simulink model "try_again_agin"  (R2025a)
settings: Solver=VariableStepAuto  StartTime=0.0  StopTime=inf  FixedStep=1e-5  MaxStep=1e-4  RelTol=1e-3
values from neighbouring files (symbols this model uses):
  B = 0.0001    [main.m]
  init_Thetar = 0    [main.m]
  init_Thetar_tilde = -3*pi/7    (= -1.34639685154)    [main.m]
  Is_rated = 10    [main.m]
  J = 0.045    [main.m]
  Kas = 1/Kps    (= 3.05577490736)    [main.m]
  Kic = Rs*Wcc    (= 1256.63706144)    [main.m]
  Kis = J*Wsc^2/5/Kt    (= 2.05616758356)    [main.m]
  Kpc = Lds*Wcc    (= 18.8495559215)    [main.m]
  Kps = J*Wsc/Kt    (= 0.327249234749)    [main.m]
  Lamf = 0.12    [main.m]
  Lds = 30.0e-3    (= 0.03)    [main.m]
  Lqs = 40.0e-3    (= 0.04)    [main.m]
  mm = 2    [main.m]
  Mode = 2    [main.m]
  P = 24    [main.m]
  Rs = 2    [main.m]
  V_inj = 60    [main.m]
  w_h = 2*pi*800    (= 5026.54824574)    [main.m]
settings Model: Creator=moon  LastModifiedBy=moon
settings RTWCC: GPUComputeCapability=3.5

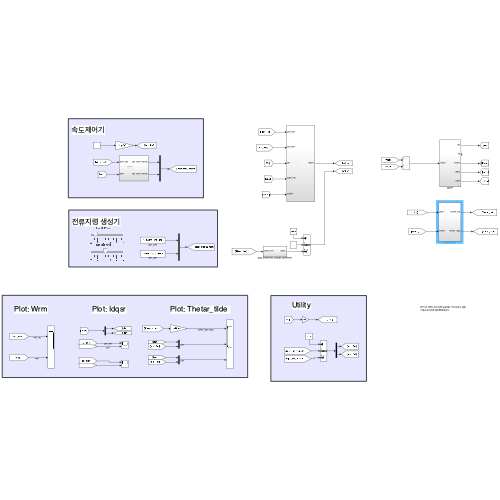
[thumbnail: Simulink's stored preview of the top-level diagram]
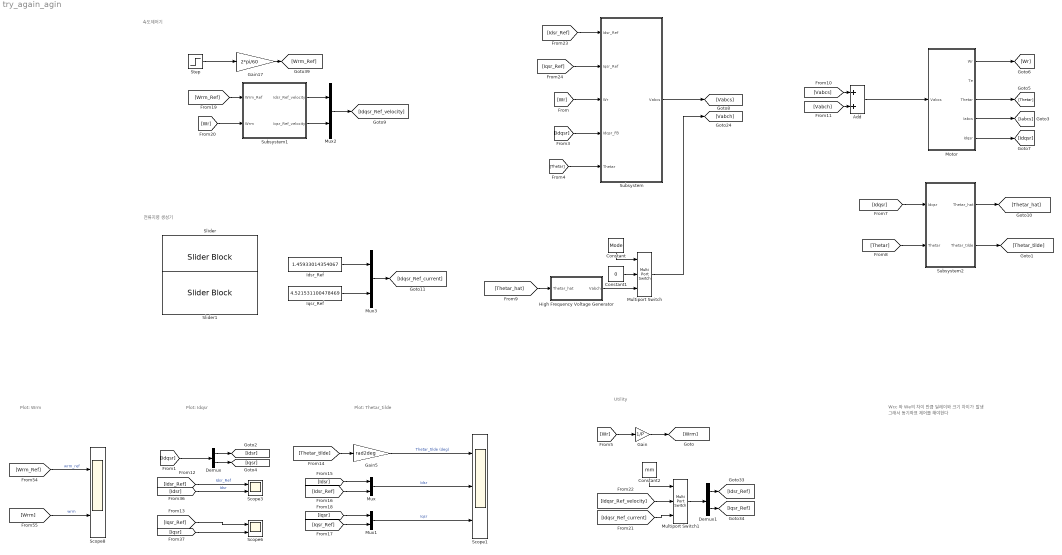
== system try_again_agin ==
  note: Plot: Thetar_tilde
  note: 전류지령 생성기
  note: 속도제어기
  note: 그래서 동기좌표 제어를 해야한다
  note: Wcc 와 We의 차이 만큼 딜레이와 크기 차이가 발생
  note: Plot: Wrm
  note: Plot: Idqsr
  note: Utility
  Add : Sum
  Constant : Constant  Value=Mode
  Constant1 : Constant  Value=0
  Constant2 : Constant  Value=mm
  Demux : Demux  Outputs=2
  Demux1 : Demux  Outputs=2
  Gain : Gain  Gain=1/P
  Gain17 : Gain  Gain=2*pi/60
  Gain5 : Gain  Gain=rad2deg
  High Frequency Voltage Generator : Subsystem
  Idsr_Ref : Constant  Value=1.45933014354067
  Iqsr_Ref : Constant  Value=4.521531100478469
  Motor : Subsystem
  Multiport Switch : MultiPortSwitch  Inputs=2  SaturateOnIntegerOverflow=off  InputSameDT=off
  Multiport Switch1 : MultiPortSwitch  Inputs=2  SaturateOnIntegerOverflow=off  InputSameDT=off
  Mux{,1..3} (4 alike) : Mux  Inputs=2
  Scope1 : Scope  NumInputPorts=3
      settings: ActiveDisplayYMinimum=-5.1750271088581092  ActiveDisplayYMaximum=6.5752439797229876  DataLoggingVariableName=ScopeData8
  Scope3 : Scope  NumInputPorts=2
      settings: ActiveDisplayYMinimum=-1  ActiveDisplayYMaximum=1  DataLoggingVariableName=ScopeData4
  Scope6 : Scope  NumInputPorts=2
      settings: ActiveDisplayYMinimum=-1.0209344961629327  ActiveDisplayYMaximum=9.1884104654663972  DataLoggingVariableName=ScopeData5
  Scope8 : Scope  NumInputPorts=2
      settings: ActiveDisplayYMinimum=-124.203723618037  ActiveDisplayYMaximum=1117.8335125623332
  Slider : SliderBlock  ScaleMax=10
  Slider1 : SliderBlock  ScaleMax=10
  Step : Step  After=200  SampleTime=0
  Subsystem : Subsystem
  Subsystem1 : Subsystem
  Subsystem2 : Subsystem
  wires:
  [Wrm_Ref] -> Scope8/1  "wrm_ref"
  [Wrm] -> Scope8/2  "wrm"
  Gain17/1 -> [Wrm_Ref]
  Step/1 -> Gain17/1
  Motor/4(Iabcs) -> [Iabcs]
  Motor/3(Thetar) -> [Thetar]
  Motor/1(Wr) -> [Wr]
  Add/1 -> Motor/1(Vabcs)
  Motor/5(Idqsr) -> [Idqsr]
  [Wr] -> Subsystem/3(Wr)
  [Idqsr] -> Subsystem/4(Idqsr_FB)
  Subsystem/1(Vabcs) -> [Vabcs]
  [Thetar] -> Subsystem/5(Thetar)
  [Wr] -> Gain/1
  Gain/1 -> [Wrm]
  [Idqsr] -> Subsystem2/1(Idqsr)
  [Thetar] -> Subsystem2/2(Thetar)
  Subsystem2/1(Thetar_hat) -> [Thetar_hat]
  Subsystem2/2(Thetar_tilde) -> [Thetar_tilde]
  [Thetar_hat] -> High Frequency Voltage Generator/1(Thetar_hat)
  High Frequency Voltage Generator/1(Vabch) -> Multiport Switch/3
  Constant1/1 -> Multiport Switch/2
  Constant/1 -> Multiport Switch/1
  [Vabch] -> Add/2
  [Vabcs] -> Add/1
  Multiport Switch/1 -> [Vabch]
  [Idsr_Ref] -> Scope3/1  "Idsr_Ref"
  [Iqsr] -> Scope6/2
  [Idsr] -> Scope3/2  "Idsr"
  [Iqsr_Ref] -> Scope6/1
  [Idqsr] -> Demux/1
  Demux/1 -> [Idsr]
  Demux/2 -> [Iqsr]
  [Idsr] -> Mux/1
  Mux/1 -> Scope1/2  "Idsr"
  Mux1/1 -> Scope1/3  "Iqsr"
  [Idsr_Ref] -> Mux/2
  Gain5/1 -> Scope1/1  "Thetar_tilde (deg)"
  [Iqsr] -> Mux1/1
  [Thetar_tilde] -> Gain5/1
  [Wrm_Ref] -> Subsystem1/1(Wrm_Ref)
  [Wr] -> Subsystem1/2(Wrm)
  Subsystem1/1(Idsr_Ref_velocity) -> Mux2/1
  Subsystem1/2(Iqsr_Ref_velocity) -> Mux2/2
  Mux2/1 -> [Idqsr_Ref_velocity]
  Iqsr_Ref/1 -> Mux3/2
  Idsr_Ref/1 -> Mux3/1
  Mux3/1 -> [Idqsr_Ref_current]
  Constant2/1 -> Multiport Switch1/1
  [Idqsr_Ref_velocity] -> Multiport Switch1/2
  [Idqsr_Ref_current] -> Multiport Switch1/3
  Multiport Switch1/1 -> Demux1/1
  Demux1/1 -> [Idsr_Ref]
  Demux1/2 -> [Iqsr_Ref]
  [Idsr_Ref] -> Subsystem/1(Idsr_Ref)
  [Iqsr_Ref] -> Subsystem/2(Iqsr_Ref)
  [Iqsr_Ref] -> Mux1/2

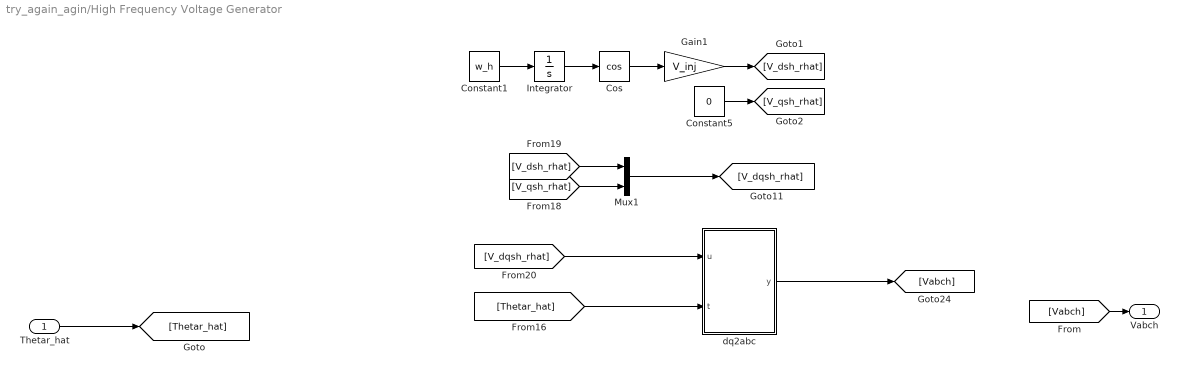
== system try_again_agin/High Frequency Voltage Generator ==
  Thetar_hat : Inport
  Constant1 : Constant  Value=w_h
  Constant5 : Constant  Value=0
  Cos : Trigonometry  Operator=cos
  Gain1 : Gain  Gain=V_inj
  Integrator : Integrator
  Mux1 : Mux  Inputs=2
  dq2abc : MATLAB Function  TreatAsAtomicUnit=on
  Vabch : Outport
  wires:
  Constant5/1 -> [V_qsh_rhat]
  Integrator/1 -> Cos/1
  Constant1/1 -> Integrator/1
  Mux1/1 -> [V_dqsh_rhat]
  Gain1/1 -> [V_dsh_rhat]
  dq2abc/1(y) -> [Vabch]
  [Thetar_hat] -> dq2abc/2(t)
  Cos/1 -> Gain1/1
  [V_dsh_rhat] -> Mux1/1
  [V_qsh_rhat] -> Mux1/2
  [V_dqsh_rhat] -> dq2abc/1(u)
  [Vabch] -> Vabch/1
  Thetar_hat/1 -> [Thetar_hat]

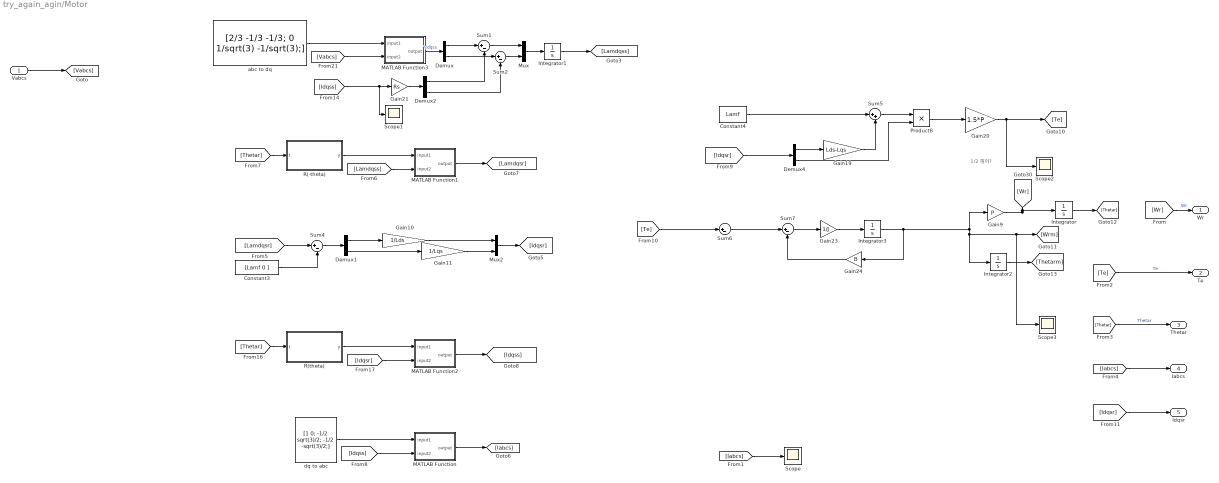
== system try_again_agin/Motor ==
  note: 1/2 해야?
  Vabcs : Inport
  Constant3 : Constant  Value=[Lamf 0 ]
  Constant4 : Constant  Value=Lamf
  Demux{,1..2,4} (4 alike) : Demux  Outputs=2
  Gain10 : Gain  Gain=1/Lds
  Gain11 : Gain  Gain=1/Lqs
  Gain19 : Gain  Gain=Lds-Lqs
  Gain20 : Gain  Gain=1.5*P
  Gain21 : Gain  Gain=Rs
  Gain23 : Gain  Gain=1/J
  Gain24 : Gain  Gain=B
  Gain9 : Gain  Gain=P
  Integrator : Integrator  InitialCondition=init_Thetar
  Integrator1 : Integrator
  Integrator2 : Integrator
  Integrator3 : Integrator
  MATLAB Function : MATLAB Function  TreatAsAtomicUnit=on
  MATLAB Function1 : MATLAB Function  TreatAsAtomicUnit=on
  MATLAB Function2 : MATLAB Function  TreatAsAtomicUnit=on
  MATLAB Function3 : MATLAB Function  TreatAsAtomicUnit=on
  Mux : Mux  Inputs=2
  Mux2 : Mux  Inputs=2
  Product8 : Product
  R(-theta) : Subsystem
      mask Display: image(imread('img/rotateInverseMatrix.png'))
  R(theta) : Subsystem
      mask Display: image(imread('img/rotateMatrix.png'))
  Scope{,1..3} (4 alike) : Scope
      Scope settings: ActiveDisplayYMinimum=-12.65498  ActiveDisplayYMaximum=12.66704
      Scope1 settings: ActiveDisplayYMinimum=-1  ActiveDisplayYMaximum=1
      Scope2 settings: ActiveDisplayYMinimum=-2.164914459316361  ActiveDisplayYMaximum=19.484230133847252  DataLoggingVariableName=ScopeData2
      Scope3 settings: ActiveDisplayYMinimum=-7240.0541502508459  ActiveDisplayYMaximum=1269.8716380292226  DataLoggingVariableName=ScopeData7
  Sum{1..2,4,6..7} (5 alike) : Sum  Inputs=|+-
  Sum5 : Sum  Inputs=|++
  abc to dq : Constant  Value=[2/3 -1/3 -1/3; 0 1/sqrt(3) -1/sqrt(3);]
      mask Display: image(imread('img/abc2dq.png'))
  dq to abc : Constant  Value=[1 0; -1/2 sqrt(3)/2; -1/2 -sqrt(3)/2;]
      mask Display: image(imread('img/dq2abc.png'))
  Wr : Outport
  Te : Outport  Port=2
  Thetar : Outport  Port=3
  Iabcs : Outport  Port=4
  Idqsr : Outport  Port=5
  wires:
  R(-theta)/1(y) -> MATLAB Function1/1(input1)
  [Idqsr] -> Demux4/1
  Product8/1 -> Gain20/1
  Sum7/1 -> Gain23/1
  Sum5/1 -> Product8/1
  [Thetar] -> R(theta)/1(t)
  [Lamdqsr] -> Sum4/1
  [Idqss] -> Scope1/1, Gain21/1
  R(theta)/1(y) -> MATLAB Function2/1(input1)
  Gain24/1 -> Sum7/2
  MATLAB Function/1(output) -> [Iabcs]
  Constant4/1 -> Sum5/1
  [Thetar] -> R(-theta)/1(t)
  MATLAB Function2/1(output) -> [Idqss]
  [Vabcs] -> MATLAB Function3/2(input2)
  Demux1/2 -> Gain11/1
  abc to dq/1 -> MATLAB Function3/1(input1)
  Gain20/1 -> Scope2/1, [Te]
  Integrator1/1 -> [Lamdqss]
  [Iabcs] -> Scope/1
  [Idqsr] -> MATLAB Function2/2(input2)
  Gain23/1 -> Integrator3/1
  Demux1/1 -> Gain10/1
  [Idqss] -> MATLAB Function/2(input2)
  Gain19/1 -> Sum5/2
  dq to abc/1 -> MATLAB Function/1(input1)
  Gain11/1 -> Mux2/2
  Demux4/2 -> Product8/2
  MATLAB Function1/1(output) -> [Lamdqsr]
  Mux2/1 -> [Idqsr]
  Constant3/1 -> Sum4/2
  Gain10/1 -> Mux2/1
  [Te] -> Sum6/1
  Integrator3/1 -> Gain24/1, Scope3/1, [Wrm], Integrator2/1, Gain9/1
  Integrator2/1 -> [Thetarm]
  Sum6/1 -> Sum7/1
  [Lamdqss] -> MATLAB Function1/2(input2)
  Sum4/1 -> Demux1/1
  Demux4/1 -> Gain19/1
  Vabcs/1 -> [Vabcs]
  [Wr] -> Wr/1  "Wr"
  [Te] -> Te/1  "Te"
  [Thetar] -> Thetar/1  "Thetar"
  [Iabcs] -> Iabcs/1
  [Idqsr] -> Idqsr/1
  MATLAB Function3/1(output) -> Demux/1  "Vdqss"
  Gain21/1 -> Demux2/1
  Sum2/1 -> Mux/2
  Sum1/1 -> Mux/1
  Demux2/1 -> Sum1/2
  Demux2/2 -> Sum2/2
  Demux/2 -> Sum2/1
  Demux/1 -> Sum1/1
  Mux/1 -> Integrator1/1
  Gain9/1 -> Integrator/1, [Wr]
  Integrator/1 -> [Thetar]

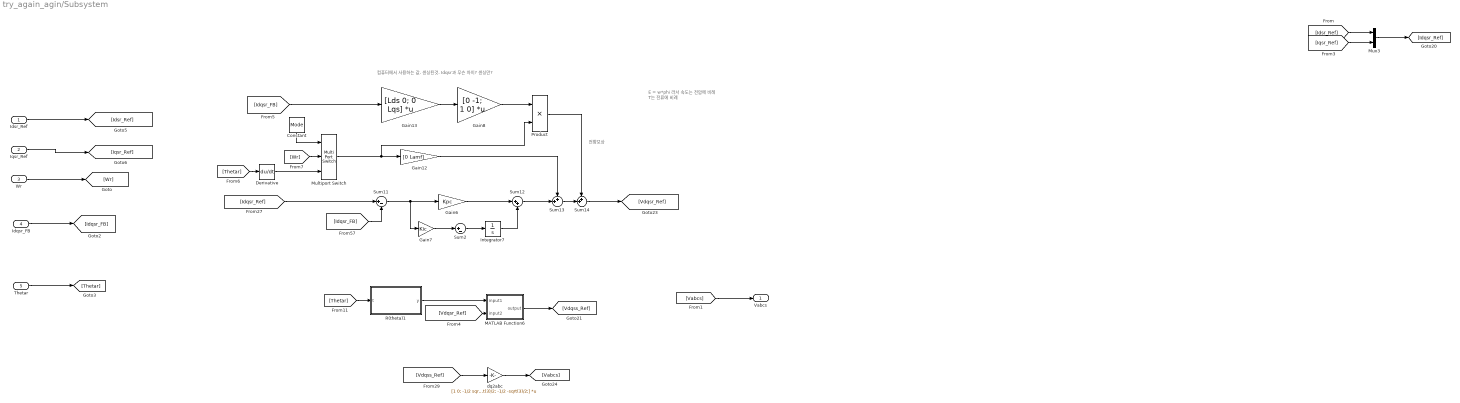
== system try_again_agin/Subsystem ==
  note: E = w*phi 라서 속도는 전압에 비례
      | T는 전류에 비례
  note: 컴퓨터에서 사용하는 값. 센싱된것. Idqsr과 무슨 차이? 센싱만?
  note: 전향보상
  Idsr_Ref : Inport
  Iqsr_Ref : Inport  Port=2
  Wr : Inport  Port=3
  Idqsr_FB : Inport  Port=4
  Thetar : Inport  Port=5
  Constant : Constant  Value=Mode
  Derivative : Derivative
  Gain12 : Gain  Gain=[0 Lamf]
  Gain13 : Gain  Gain=[Lds 0; 0 Lqs]  Multiplication=Matrix(K*u)
  Gain6 : Gain  Gain=Kpc
  Gain7 : Gain  Gain=Kic
  Gain8 : Gain  Gain=[0 -1; 1 0]  Multiplication=Matrix(K*u)
  Integrator7 : Integrator
  MATLAB Function6 : MATLAB Function  TreatAsAtomicUnit=on
  Multiport Switch : MultiPortSwitch  Inputs=2  SaturateOnIntegerOverflow=off  InputSameDT=off
  Mux3 : Mux  Inputs=2
  Product : Product
  R(theta)1 : Subsystem
      mask Display: image(imread('img/rotateMatrix.png'))
  Sum11 : Sum  Inputs=|+-
  Sum12 : Sum  Inputs=|++
  Sum13 : Sum  Inputs=++|
  Sum14 : Sum  Inputs=++|
  Sum2 : Sum  Inputs=|+-
  dq2abc : Gain  Gain=[1 0; -1/2 sqrt(3)/2; -1/2 -sqrt(3)/2;]  Multiplication=Matrix(K*u)
  Vabcs : Outport
  wires:
  Product/1 -> Sum14/1
  [Thetar] -> R(theta)1/1(t)
  [Iqsr_Ref] -> Mux3/2
  [Idsr_Ref] -> Mux3/1
  [Idqsr_FB] -> Gain13/1
  R(theta)1/1(y) -> MATLAB Function6/1(input1)
  Gain13/1 -> Gain8/1
  MATLAB Function6/1(output) -> [Vdqss_Ref]
  Sum13/1 -> Sum14/2
  [Idqsr_FB] -> Sum11/2
  Integrator7/1 -> Sum12/2
  Gain8/1 -> Product/1
  Gain6/1 -> Sum12/1
  Multiport Switch/1 -> Product/2, Gain12/1
  [Idqsr_Ref] -> Sum11/1
  Mux3/1 -> [Idqsr_Ref]
  Gain12/1 -> Sum13/1
  Sum11/1 -> Gain6/1, Gain7/1
  [Vdqsr_Ref] -> MATLAB Function6/2(input2)
  Sum12/1 -> Sum13/2
  Wr/1 -> [Wr]
  Idqsr_FB/1 -> [Idqsr_FB]
  [Vabcs] -> Vabcs/1
  Thetar/1 -> [Thetar]
  Gain7/1 -> Sum2/1
  Sum2/1 -> Integrator7/1
  [Vdqss_Ref] -> dq2abc/1
  dq2abc/1 -> [Vabcs]
  Sum14/1 -> [Vdqsr_Ref]
  Derivative/1 -> Multiport Switch/3
  Constant/1 -> Multiport Switch/1
  [Thetar] -> Derivative/1
  [Wr] -> Multiport Switch/2
  Idsr_Ref/1 -> [Idsr_Ref]
  Iqsr_Ref/1 -> [Iqsr_Ref]

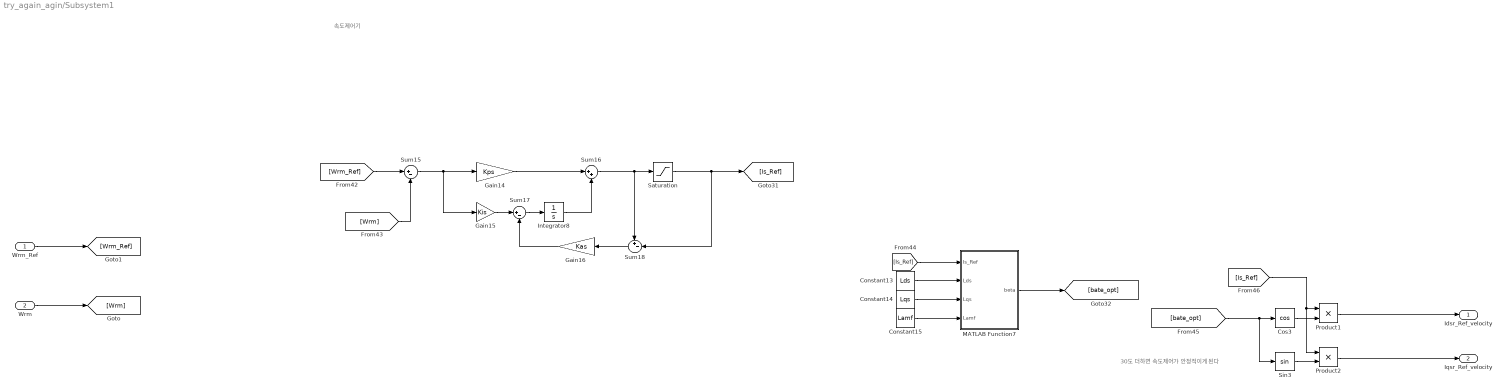
== system try_again_agin/Subsystem1 ==
  note: 30도 더하면 속도제어가 안정적이게 된다
  note: 속도제어기
  Wrm_Ref : Inport
  Wrm : Inport  Port=2
  Constant13 : Constant  Value=Lds
  Constant14 : Constant  Value=Lqs
  Constant15 : Constant  Value=Lamf
  Cos3 : Trigonometry  Operator=cos
  Gain14 : Gain  Gain=Kps
  Gain15 : Gain  Gain=Kis
  Gain16 : Gain  Gain=Kas
  Integrator8 : Integrator
  MATLAB Function7 : MATLAB Function  TreatAsAtomicUnit=on
  Product1 : Product
  Product2 : Product
  Saturation : Saturate  UpperLimit=Is_rated  LowerLimit=-Is_rated
  Sin3 : Trigonometry
  Sum15 : Sum  Inputs=|+-
  Sum16 : Sum  Inputs=|++
  Sum17 : Sum  Inputs=|+-
  Sum18 : Sum  Inputs=+-|
  Idsr_Ref_velocity : Outport
  Iqsr_Ref_velocity : Outport  Port=2
  wires:
  Gain15/1 -> Sum17/1
  [Wrm_Ref] -> Sum15/1
  Saturation/1 -> [Is_Ref], Sum18/2
  Gain16/1 -> Sum17/2
  Sum16/1 -> Saturation/1, Sum18/1
  Product2/1 -> Iqsr_Ref_velocity/1
  Gain14/1 -> Sum16/1
  Product1/1 -> Idsr_Ref_velocity/1
  [Wrm] -> Sum15/2
  Constant14/1 -> MATLAB Function7/3(Lqs)
  [Is_Ref] -> MATLAB Function7/1(Is_Ref)
  Constant13/1 -> MATLAB Function7/2(Lds)
  MATLAB Function7/1(beta) -> [bate_opt]
  Sum18/1 -> Gain16/1
  Sum15/1 -> Gain15/1, Gain14/1
  [Is_Ref] -> Product2/1, Product1/1
  Cos3/1 -> Product1/2
  Sum17/1 -> Integrator8/1
  [bate_opt] -> Cos3/1, Sin3/1
  Sin3/1 -> Product2/2
  Integrator8/1 -> Sum16/2
  Constant15/1 -> MATLAB Function7/4(Lamf)
  Wrm/1 -> [Wrm]
  Wrm_Ref/1 -> [Wrm_Ref]

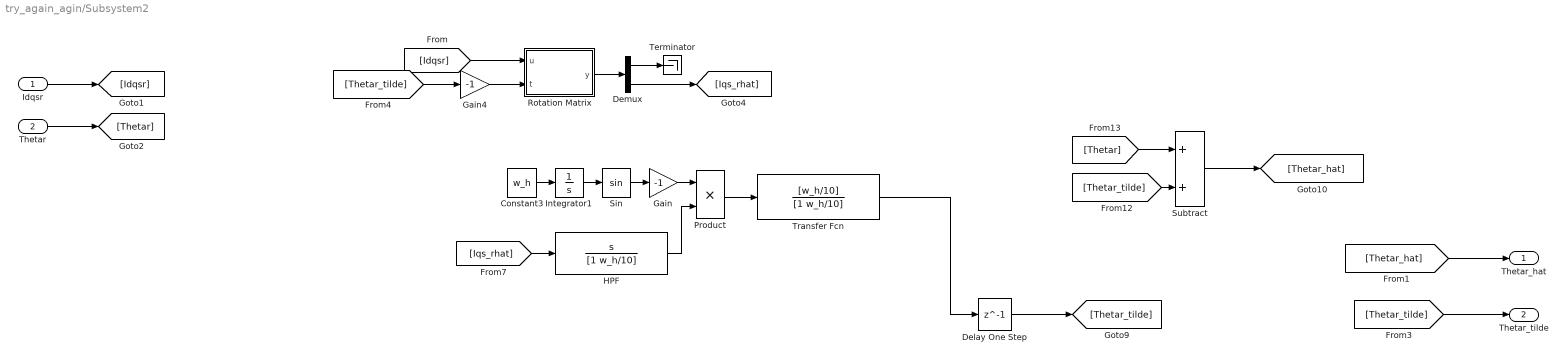
== system try_again_agin/Subsystem2 ==
  Idqsr : Inport
  Thetar : Inport  Port=2
  Constant3 : Constant  Value=w_h
  Delay One Step : Delay  DelayLength=1  InitialCondition=init_Thetar_tilde
  Demux : Demux  Outputs=2
  Gain : Gain  Gain=-1
  Gain4 : Gain  Gain=-1
  HPF : TransferFcn  Numerator=[1 0]  Denominator=[1 w_h/10]
  Integrator1 : Integrator
  Product : Product
  Rotation Matrix : MATLAB Function  TreatAsAtomicUnit=on
  Sin : Trigonometry
  Subtract : Sum
  Terminator : Terminator
  Transfer Fcn : TransferFcn  Numerator=[w_h/10]  Denominator=[1 w_h/10]
  Thetar_hat : Outport
  Thetar_tilde : Outport  Port=2
  wires:
  Subtract/1 -> [Thetar_hat]
  Product/1 -> Transfer Fcn/1
  Constant3/1 -> Integrator1/1
  Demux/2 -> [Iqs_rhat]
  Rotation Matrix/1(y) -> Demux/1
  Gain4/1 -> Rotation Matrix/2(t)
  [Iqs_rhat] -> HPF/1
  Integrator1/1 -> Sin/1
  HPF/1 -> Product/2
  [Thetar_tilde] -> Subtract/2
  Transfer Fcn/1 -> Delay One Step/1
  Demux/1 -> Terminator/1
  [Thetar] -> Subtract/1
  Sin/1 -> Gain/1
  [Thetar_tilde] -> Gain4/1
  [Idqsr] -> Rotation Matrix/1(u)
  Idqsr/1 -> [Idqsr]
  Thetar/1 -> [Thetar]
  [Thetar_hat] -> Thetar_hat/1
  Gain/1 -> Product/1
  [Thetar_tilde] -> Thetar_tilde/1
  Delay One Step/1 -> [Thetar_tilde]

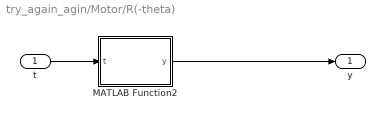
== system try_again_agin/Motor/R(-theta) ==
  t : Inport
  MATLAB Function2 : MATLAB Function  TreatAsAtomicUnit=on
  y : Outport
  wires:
  MATLAB Function2/1(y) -> y/1
  t/1 -> MATLAB Function2/1(t)

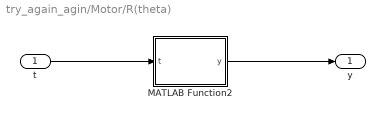
== system try_again_agin/Motor/R(theta) ==
  t : Inport
  MATLAB Function2 : MATLAB Function  TreatAsAtomicUnit=on
  y : Outport
  wires:
  MATLAB Function2/1(y) -> y/1
  t/1 -> MATLAB Function2/1(t)

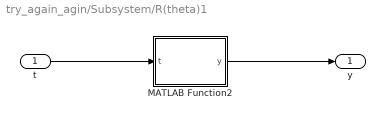
== system try_again_agin/Subsystem/R(theta)1 ==
  t : Inport
  MATLAB Function2 : MATLAB Function  TreatAsAtomicUnit=on
  y : Outport
  wires:
  MATLAB Function2/1(y) -> y/1
  t/1 -> MATLAB Function2/1(t)

== matlab function try_again_agin/Motor/MATLAB Function1 ==
  data: input1 input; output output; input2 input
function output = matrix_multiply(input1, input2)
    % 행렬 곱셈 (input1의 열 수 = input2의 행 수)
    output = input1 * input2;
end

== matlab function try_again_agin/Motor/MATLAB Function ==
  data: input1 input; output output; input2 input
function output = matrix_multiply(input1, input2)
    % 행렬 곱셈 (input1의 열 수 = input2의 행 수)
    output = input1 * input2;
end

== matlab function try_again_agin/Motor/R(-theta)/MATLAB Function2 ==
  data: t input; y output
function y = matrix_output(t)
y = [cos(t) sin(t); -sin(t) cos(t)];

== matlab function try_again_agin/Motor/MATLAB Function2 ==
  data: input1 input; output output; input2 input
function output = matrix_multiply(input1, input2)
    % 행렬 곱셈 (input1의 열 수 = input2의 행 수)
    output = input1 * input2;
end

== matlab function try_again_agin/Motor/R(theta)/MATLAB Function2 ==
  data: t input; y output
function y = matrix_output(t)
y = [cos(t) -sin(t); sin(t) cos(t)];

== matlab function try_again_agin/Motor/MATLAB Function3 ==
  data: input1 input; output output; input2 input
function output = matrix_multiply(input1, input2)
    % 행렬 곱셈 (input1의 열 수 = input2의 행 수)
    output = input1 * input2;
end

== matlab function try_again_agin/Subsystem2/Rotation Matrix ==
  data: u input size=[2 1]; y output size=[2 1]; t input
function y = fcn(u, t)

R = [cos(t) -sin(t); sin(t) cos(t)];

y = R*u;

== matlab function try_again_agin/Subsystem/MATLAB Function6 ==
  data: input1 input; output output; input2 input
function output = matrix_multiply(input1, input2)
    % 행렬 곱셈 (input1의 열 수 = input2의 행 수)
    output = input1 * input2;
end

== matlab function try_again_agin/Subsystem/R(theta)1/MATLAB Function2 ==
  data: t input; y output
function y = matrix_output(t)
y = [cos(t) -sin(t); sin(t) cos(t)];

== matlab function try_again_agin/Subsystem1/MATLAB Function7 ==
  data: Is_Ref input; beta output; Lds input; Lqs input; Lamf input
function beta = fcn(Is_Ref, Lds, Lqs, Lamf)

beta = acos((-Lamf+sqrt(Lamf^2+8*(Lds-Lqs)^2*Is_Ref^2))/(4*(Lds-Lqs)*(Is_Ref+0.001)));

== matlab function try_again_agin/High Frequency Voltage Generator/dq2abc ==
  data: u input size=[2 1]; y output size=[3 1]; t input
function y = fcn(u, t)

a=2*pi/3;

TT = @(t) ...
    [cos(t)  cos(t-a)  cos(t+a);
    -sin(t) -sin(t-a) -sin(t+a);
        1/2       1/2       1/2;] *2/3;

y = TT(t) \ [u; 0];
